simulink model "ADIA"  (R2018b)
settings: Solver=FixedStepDiscrete  StartTime=0.0  StopTime=10.0  FixedStep=0.02  RelTol=1e-3
undefined symbols (not defined in the file or in its folder): ACC_State_Active, ACC_State_BrakeOnly, ACC_State_Suspended, ACC_State_WaitingRise, ADAS_AEBBrakingProg, ADAS_DeclControlReq, ADAS_DriveOff, ADAS_ESCHoldReq_NotHold, ADASDecType_ACC, ADASDecType_AEB, ADIA_ACC_Acceleration_OOR_DecCount_C, ADIA_ACC_Acceleration_OOR_Duration_C, ADIA_ACC_Acceleration_OOR_IncCount_C, ADIA_ACC_Acceleration_OOR_LLim_C, ADIA_ACC_Acceleration_OOR_ULim_C, ADIA_ACC_AccelTrqReq_MixedDia_ULim_C, ADIA_ACC_AccelTrqReq_ULim_C, ADIA_ACC_Deceleration_Mixed_ULim_C, ADIA_ACC_Deceleration_OOR_DecCount_C, ADIA_ACC_Deceleration_OOR_Duration_C, ADIA_ACC_Deceleration_OOR_IncCount_C, ADIA_ACC_Deceleration_OOR_LLim_C, ADIA_ACC_Deceleration_OOR_ULim_C, ADIA_ACC_DriveOff_Distance_C, ADIA_ACC_DriveOff_TimeLim_C, ADIA_ACC_ReqMixed_DecCount_C, ADIA_ACC_ReqMixed_Duration_C, ADIA_ACC_ReqMixed_IncCount_C, ADIA_AccPedalRaw_MaxLim_C, ADIA_AccPedalRaw_MinLim_C, ADIA_ADAS_HoldDecReq_Set_C, ADIA_ADAS_HoldRConfirm_TimeLim_C, ADIA_ADAS_HoldVehSpd_Lim_C, ADIA_AEB_VehSpdDec_LLim_C, ADIA_AEB_VehSpdDec_ULim_C, ADIA_ASWFault_OvrdEn_C, ADIA_ASWFault_OvrdValue_C, ADIA_BatteryOutOfRange_DecCount_C, ADIA_BatteryOutOfRange_Duration_C, ADIA_BatteryOutOfRange_IncCount_C, ADIA_BattVolt_MaxLim_C, ADIA_BattVolt_MinLim_C, ADIA_BCM3_33C_InvBrkLight_DecCount_C, ADIA_BCM3_33C_InvBrkLight_Duration_C, ADIA_BCM3_33C_InvBrkLight_IncCount_C, ADIA_BCM_BattVolt_OvrdEn_C, ADIA_BCM_BattVolt_OvrdVal_C, ADIA_BCM_BrakeLampStaus_OvrdEn_C, ADIA_BCM_BrakeLampStaus_OvrdVal_C, ADIA_BCM_CHMSLStaus_OvrdEn_C, ADIA_BCM_CHMSLStaus_OvrdVal_C, ADIA_BCM_LeftTurnSwSt_OvrdEn_C, ADIA_BCM_LeftTurnSwSt_OvrdVal_C, ADIA_BCM_RightTurnSwSt_OvrdEn_C, ADIA_BCM_RightTurnSwSt_OvrdVal_C, ADIA_BCM_TurnSwFailure_DecCount_C, ADIA_BCM_TurnSwFailure_Duration_C, ADIA_BCM_TurnSwFailure_IncCount_C, ADIA_BSWFault_Ignore_C, ADIA_BSWFault_OvrdEn_C ... (+281)
libraries: simulink x208
(part 4 of 10)

== system ADIA/ADAS_Diagnostics/Diagnostics_Processing/DTC_ACC_Displacement_Safety_Violation ==
  note: may have some reset question
  ADIAve_y_ADAS_ESCDriveOff : Inport  OutDataTypeStr=UInt8  PortDimensions=1
  ADIAve_y_ADAS_ESCHoldReq : Inport  Port=2  OutDataTypeStr=UInt8  PortDimensions=1
  ADIAve_y_ADAS_ACCState : Inport  Port=3  OutDataTypeStr=UInt8  PortDimensions=1
  ADIAve_g_ESC_VehSpd : Inport  Port=4  OutDataTypeStr=single  PortDimensions=1
  Constant1 : Constant  Value=SYS_dT20ms
  Constant11 : Constant  Value=ADIA_ACC_DriveOff_TimeLim_C
  Constant12 : Constant  Value=ADIA_ACC_DriveOff_Distance_C
  Constant2 : Constant  Value=mps_to_kph  OutDataTypeStr=Inherit: Inherit via back propagation
  Constant3 : Constant  Value=ADAS_DriveOff
  Constant4 : Constant  Value=SYS_dT20ms
  Constant5 : Constant  Value=SYS_False
  Constant6 : Constant  Value=0
  Constant7 : Constant  Value=ADAS_ESCHoldReq_NotHold
  Constant9 : Constant  Value=ACC_State_Active  OutDataTypeStr=Inherit: Inherit via back propagation
  Counter : Subsystem
  Divide : Product  Inputs=*/
  Divide1 : Product  Inputs=**
  Latch 2 : Subsystem
  Logical Operator{1,3,7..8} (4 alike) : Logic  Operator=NOT  AllPortsSameDT=off  OutDataTypeStr=boolean
  Logical Operator{2,4..6} (4 alike) : Logic  AllPortsSameDT=off  OutDataTypeStr=boolean
  Relational Operator1 : RelationalOperator  Operator===  OutDataTypeStr=boolean  RndMeth=Simplest
  Relational Operator5 : RelationalOperator  Operator===  OutDataTypeStr=boolean  RndMeth=Simplest
  Relational Operator7 : RelationalOperator  Operator===  OutDataTypeStr=boolean  RndMeth=Simplest
  Terminator : Terminator
  Terminator1 : Terminator
  Timer1 : Subsystem
  ADIA_DTC_ACC_Displacement_Safety_Violation : Outport
  wires:
  ADIAve_y_ADAS_ESCHoldReq/1 -> Relational Operator5/1
  Constant7/1 -> Relational Operator5/2
  Relational Operator5/1 -> Logical Operator4/2
  Constant9/1 -> Relational Operator7/2
  ADIAve_y_ADAS_ACCState/1 -> Relational Operator7/1
  Relational Operator7/1 -> Logical Operator5/1
  Logical Operator5/1 -> Logical Operator3/1, Logical Operator2/2, Timer1/1(incrcondition)
  Constant12/1 -> Counter/2(maxlimit)
  Counter/2(counter_status) -> Logical Operator8/1, Latch 2/1(Input)
  Counter/1(counter out) -> Terminator/1
  Latch 2/1(Output) -> ADIA_DTC_ACC_Displacement_Safety_Violation/1
  ADIAve_g_ESC_VehSpd/1 -> Divide/1
  Constant2/1 -> Divide/2
  ADIAve_y_ADAS_ESCDriveOff/1 -> Relational Operator1/1
  Constant3/1 -> Relational Operator1/2
  Logical Operator4/1 -> Logical Operator5/2
  Relational Operator1/1 -> Logical Operator4/1
  Divide/1 -> Divide1/1
  Divide1/1 -> Counter/1(ADIAve_g_ESC_VeSpd)
  Constant4/1 -> Divide1/2
  Constant1/1 -> Timer1/2(incrvalue)
  Constant5/1 -> Timer1/3(decr condition)
  Constant6/1 -> Timer1/4(decvalue)
  Constant11/1 -> Timer1/5(maxlimit)
  Timer1/2(counter_status) -> Logical Operator1/1
  Logical Operator2/1 -> Logical Operator7/1, Counter/Enable
  Logical Operator1/1 -> Logical Operator2/1
  Timer1/1(counter out) -> Terminator1/1
  Logical Operator3/1 -> Timer1/6(reset)
  Logical Operator7/1 -> Logical Operator6/1
  Logical Operator6/1 -> Latch 2/2(Latch Reset)
  Logical Operator8/1 -> Logical Operator6/2

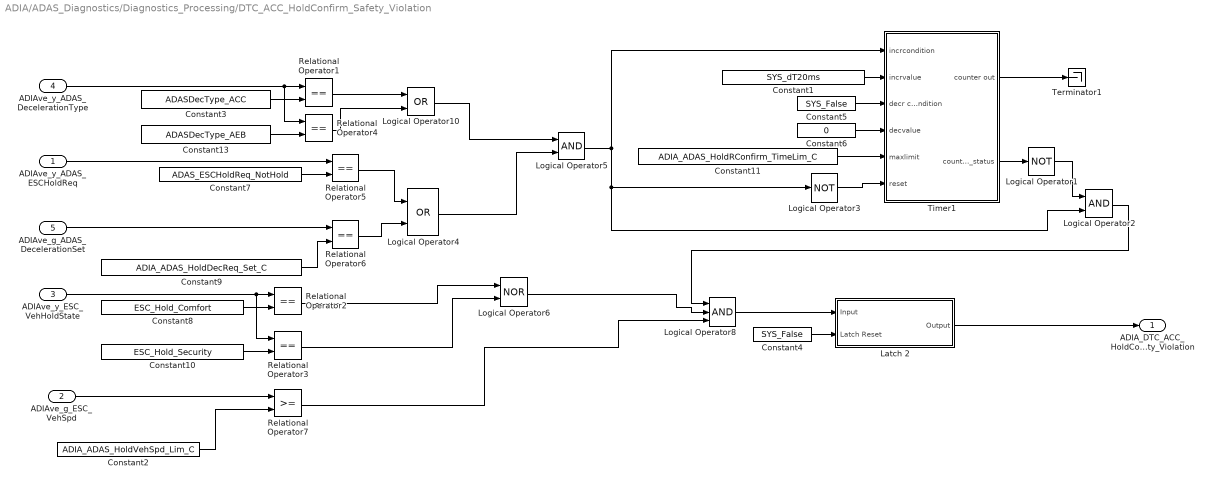
== system ADIA/ADAS_Diagnostics/Diagnostics_Processing/DTC_ACC_HoldConfirm_Safety_Violation ==
  ADIAve_y_ADAS_ESCHoldReq : Inport  OutDataTypeStr=UInt8  PortDimensions=1
  ADIAve_g_ESC_VehSpd : Inport  Port=2  OutDataTypeStr=single  PortDimensions=1
  ADIAve_y_ESC_VehHoldState : Inport  Port=3  OutDataTypeStr=uint8  PortDimensions=1
  ADIAve_y_ADAS_DecelerationType : Inport  Port=4  OutDataTypeStr=UInt8  PortDimensions=1
  ADIAve_g_ADAS_DecelerationSet : Inport  Port=5  OutDataTypeStr=T_M_Nm_Float32  PortDimensions=1
  Constant1 : Constant  Value=SYS_dT20ms
  Constant10 : Constant  Value=ESC_Hold_Security
  Constant11 : Constant  Value=ADIA_ADAS_HoldRConfirm_TimeLim_C
  Constant13 : Constant  Value=ADASDecType_AEB
  Constant2 : Constant  Value=ADIA_ADAS_HoldVehSpd_Lim_C
  Constant3 : Constant  Value=ADASDecType_ACC
  Constant4 : Constant  Value=SYS_False
  Constant5 : Constant  Value=SYS_False
  Constant6 : Constant  Value=0
  Constant7 : Constant  Value=ADAS_ESCHoldReq_NotHold
  Constant8 : Constant  Value=ESC_Hold_Comfort
  Constant9 : Constant  Value=ADIA_ADAS_HoldDecReq_Set_C
  Latch 2 : Subsystem
  Logical Operator1 : Logic  Operator=NOT  AllPortsSameDT=off  OutDataTypeStr=boolean
  Logical Operator10 : Logic  Operator=OR  AllPortsSameDT=off  OutDataTypeStr=boolean
  Logical Operator2 : Logic  AllPortsSameDT=off  OutDataTypeStr=boolean
  Logical Operator3 : Logic  Operator=NOT  AllPortsSameDT=off  OutDataTypeStr=boolean
  Logical Operator4 : Logic  Operator=OR  AllPortsSameDT=off  OutDataTypeStr=boolean
  Logical Operator5 : Logic  AllPortsSameDT=off  OutDataTypeStr=boolean
  Logical Operator6 : Logic  Operator=NOR  AllPortsSameDT=off  OutDataTypeStr=boolean
  Logical Operator8 : Logic  Inputs=3  AllPortsSameDT=off  OutDataTypeStr=boolean
  Relational Operator{1..6} (6 alike) : RelationalOperator  Operator===  OutDataTypeStr=boolean  RndMeth=Simplest
  Relational Operator7 : RelationalOperator  OutDataTypeStr=boolean  RndMeth=Simplest
  Terminator1 : Terminator
  Timer1 : Subsystem
  ADIA_DTC_ACC_HoldConfirm_Safety_Violation : Outport
  wires:
  Logical Operator3/1 -> Timer1/6(reset)
  Timer1/1(counter out) -> Terminator1/1
  Logical Operator1/1 -> Logical Operator2/1
  Logical Operator2/1 -> Logical Operator8/1
  Timer1/2(counter_status) -> Logical Operator1/1
  Constant11/1 -> Timer1/5(maxlimit)
  Constant6/1 -> Timer1/4(decvalue)
  Constant5/1 -> Timer1/3(decr condition)
  Constant1/1 -> Timer1/2(incrvalue)
  Logical Operator4/1 -> Logical Operator5/2
  Constant2/1 -> Relational Operator7/2
  ADIAve_g_ESC_VehSpd/1 -> Relational Operator7/1
  Latch 2/1(Output) -> ADIA_DTC_ACC_HoldConfirm_Safety_Violation/1
  Logical Operator5/1 -> Timer1/1(incrcondition), Logical Operator2/2, Logical Operator3/1
  Relational Operator5/1 -> Logical Operator4/1
  Constant7/1 -> Relational Operator5/2
  ADIAve_y_ADAS_ESCHoldReq/1 -> Relational Operator5/1
  ADIAve_y_ESC_VehHoldState/1 -> Relational Operator3/1, Relational Operator2/1
  Constant8/1 -> Relational Operator2/2
  Constant10/1 -> Relational Operator3/2
  Relational Operator3/1 -> Logical Operator6/2
  ADIAve_y_ADAS_DecelerationType/1 -> Relational Operator4/1, Relational Operator1/1
  Constant3/1 -> Relational Operator1/2
  Constant13/1 -> Relational Operator4/2
  Relational Operator1/1 -> Logical Operator10/1
  Relational Operator4/1 -> Logical Operator10/2
  ADIAve_g_ADAS_DecelerationSet/1 -> Relational Operator6/1
  Constant9/1 -> Relational Operator6/2
  Relational Operator6/1 -> Logical Operator4/2
  Logical Operator10/1 -> Logical Operator5/1
  Relational Operator2/1 -> Logical Operator6/1
  Relational Operator7/1 -> Logical Operator8/3
  Logical Operator6/1 -> Logical Operator8/2
  Logical Operator8/1 -> Latch 2/1(Input)
  Constant4/1 -> Latch 2/2(Latch Reset)

== system ADIA/ADAS_Diagnostics/Diagnostics_Processing/DTC_ACC_Mixed_Mode_Conflict ==
  ADIAve_y_ADAS_ACCState : Inport  OutDataTypeStr=UInt8  PortDimensions=1
  ADIAve_y_ADAS_DecelerationType : Inport  Port=2  OutDataTypeStr=UInt8  PortDimensions=1
  ADIAve_g_ADAS_ACCTorqueReq : Inport  Port=3  OutDataTypeStr=T_M_Nm_Float32  PortDimensions=1
  ADIAve_g_ADAS_DecelerationSet : Inport  Port=4  OutDataTypeStr=T_M_Nm_Float32  PortDimensions=1
  Constant : Constant  Value=ACC_State_Active
  Constant1 : Constant  Value=ACC_State_Suspended
  Constant2 : Constant  Value=ACC_State_WaitingRise
  Constant7 : Constant  Value=ACC_State_BrakeOnly
  Logical Operator4 : Logic  Operator=OR  Inputs=4  AllPortsSameDT=off  OutDataTypeStr=boolean
  Relational Operator{,1..2,5} (4 alike) : RelationalOperator  Operator===  OutDataTypeStr=boolean  RndMeth=Simplest
  Subsystem : Subsystem
  ADIA_DTC_ACC_Mixed_Mode_Conflict : Outport
  wires:
  Relational Operator5/1 -> Logical Operator4/2
  Constant7/1 -> Relational Operator5/2
  Relational Operator/1 -> Logical Operator4/1
  ADIAve_y_ADAS_ACCState/1 -> Relational Operator/1, Relational Operator2/1, Relational Operator1/1, Relational Operator5/1
  Constant/1 -> Relational Operator/2
  ADIAve_y_ADAS_DecelerationType/1 -> Subsystem/1(ADIAve_y_ADAS_DecelerationType)
  ADIAve_g_ADAS_ACCTorqueReq/1 -> Subsystem/2(ADIAve_g_ADAS_ACCTorqueReq)
  ADIAve_g_ADAS_DecelerationSet/1 -> Subsystem/3(ADIAve_g_ADAS_DecelerationSet)
  Subsystem/1(ADIA_DTC_ACC_Mixed_Mode_Conflic) -> ADIA_DTC_ACC_Mixed_Mode_Conflict/1
  Logical Operator4/1 -> Subsystem/Enable
  Constant1/1 -> Relational Operator1/2
  Relational Operator1/1 -> Logical Operator4/3
  Constant2/1 -> Relational Operator2/2
  Relational Operator2/1 -> Logical Operator4/4

== system ADIA/ADAS_Diagnostics/Diagnostics_Processing/DTC_AEB_Safety_Violation ==
  ADIAve_g_ESC_VehSpd : Inport  OutDataTypeStr=single  PortDimensions=1
  ADIAve_y_ADAS_DecelerationType : Inport  Port=2  OutDataTypeStr=UInt8  PortDimensions=1
  ADIAve_y_ADAS_DeclControlReq : Inport  Port=3  OutDataTypeStr=UInt8  PortDimensions=1
  ADIAve_y_ADAS_AEBBrakingProg : Inport  Port=4  OutDataTypeStr=UInt8  PortDimensions=1
  Add : Sum  Inputs=+-
  Constant1 : Constant  Value=ADIA_AEB_VehSpdDec_LLim_C
  Constant13 : Constant  Value=ADASDecType_AEB
  Constant2 : Constant  Value=ADIA_AEB_VehSpdDec_ULim_C
  Constant3 : Constant  Value=ADAS_AEBBrakingProg
  Constant7 : Constant  Value=ADAS_DeclControlReq
  Latch 1 : Subsystem
  Logical Operator1 : Logic  Operator=NOT  AllPortsSameDT=off  OutDataTypeStr=boolean
  Logical Operator2 : Logic  AllPortsSameDT=off  OutDataTypeStr=boolean
  Logical Operator3 : Logic  Operator=NOT  AllPortsSameDT=off  OutDataTypeStr=boolean
  Logical Operator4 : Logic  Inputs=3  AllPortsSameDT=off  OutDataTypeStr=boolean
  Logical Operator5 : Logic  AllPortsSameDT=off  OutDataTypeStr=boolean
  Relational Operator : RelationalOperator  Operator=>  OutDataTypeStr=boolean  RndMeth=Simplest
  Relational Operator1 : RelationalOperator  Operator===  OutDataTypeStr=boolean  RndMeth=Simplest
  Relational Operator2 : RelationalOperator  Operator=<=  OutDataTypeStr=boolean  RndMeth=Simplest
  Relational Operator4 : RelationalOperator  Operator===  OutDataTypeStr=boolean  RndMeth=Simplest
  Relational Operator5 : RelationalOperator  Operator===  OutDataTypeStr=boolean  RndMeth=Simplest
  Subsystem : Subsystem
  Subsystem1 : Subsystem
  Unit Delay : UnitDelay  SampleTime=-1
  Unit Delay1 : UnitDelay  SampleTime=-1
  DTC_AEB_Safety_Violation : Outport
  wires:
  Constant13/1 -> Relational Operator4/2
  ADIAve_y_ADAS_DecelerationType/1 -> Relational Operator4/1
  ADIAve_y_ADAS_DeclControlReq/1 -> Relational Operator5/1
  Constant7/1 -> Relational Operator5/2
  ADIAve_g_ESC_VehSpd/1 -> Subsystem1/1(ADIAve_g_ESC_VeSpd), Subsystem/1(ADIAve_g_ESC_VeSpd)
  Logical Operator4/1 -> Logical Operator3/1, Unit Delay1/1, Unit Delay/1, Logical Operator5/1
  Constant3/1 -> Relational Operator1/2
  ADIAve_y_ADAS_AEBBrakingProg/1 -> Relational Operator1/1
  Relational Operator1/1 -> Logical Operator4/3
  Relational Operator5/1 -> Logical Operator4/2
  Relational Operator4/1 -> Logical Operator4/1
  Logical Operator1/1 -> Logical Operator5/2
  Unit Delay/1 -> Logical Operator1/1
  Logical Operator5/1 -> Subsystem/Enable
  Unit Delay1/1 -> Logical Operator2/1
  Logical Operator3/1 -> Logical Operator2/2
  Logical Operator2/1 -> Subsystem1/Enable
  Subsystem/1(ADIA_AEB_Begin_VehSpd) -> Add/1
  Subsystem1/1(ADIA_AEB_End_VehSpd) -> Add/2
  Add/1 -> Relational Operator2/1, Relational Operator/1
  Constant2/1 -> Relational Operator/2
  Relational Operator/1 -> Latch 1/1(Input)
  Relational Operator2/1 -> Latch 1/2(Latch Reset)
  Latch 1/1(Output) -> DTC_AEB_Safety_Violation/1
  Constant1/1 -> Relational Operator2/2

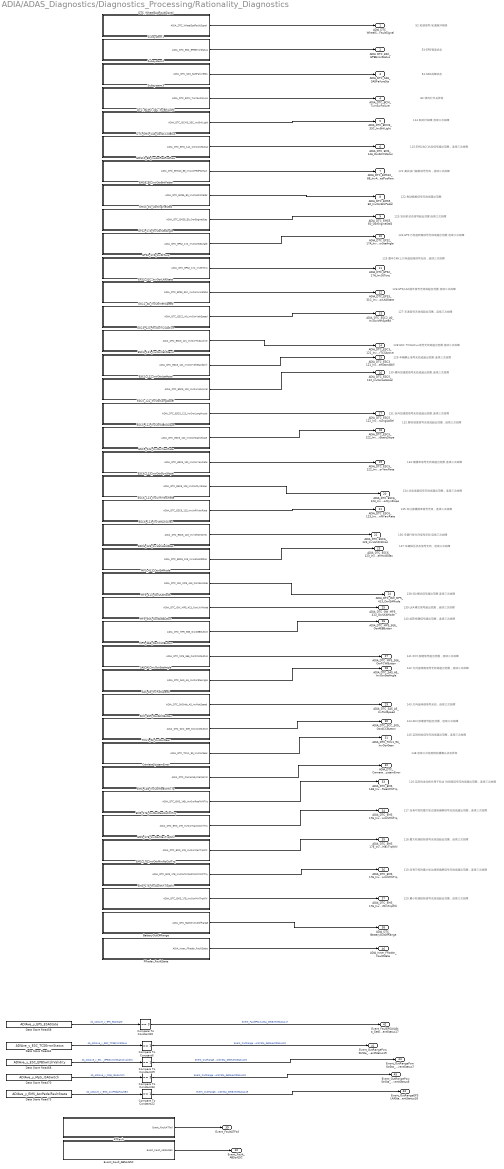
== system ADIA/ADAS_Diagnostics/Diagnostics_Processing/Rationality_Diagnostics ==
  note: 52:轮速信号/轮速脉冲错误
  note: 53:EPB错误状态
  note: 54:SAS故障状态
  note: 82:转向灯开关异常
  note: 114:制动灯故障,连续三次故障
  note: 115:EMS/ACC状态信号超出范围，连续三次故障
  note: 116:实际的发动机作用于轮边 的扭矩信号无效或超出范围，连续三次故障
  note: 117:没有可控的最大轮边扭矩偏移信号无效或超出范围，连续三次故障
  note: 118:最大轮端扭矩信号无效或超出范围，连续三次故障
  note: 119:没有可控的最小轮边扭矩偏移信号无效或超出范围，连续三次故障
  note: 120:最小轮端扭矩信号无效或超出范围，连续三次故障
  note: 121:真实油门踏板信号无效，连续三次故障
  note: 122:制动踏板信号无效或超出范围
  note: 123:发动机状态信号超出范围,连续三次故障
  note: 124:EPS 方向盘转角信号无效或超出范围,连续三次故障
  note: 125:整车CAN上方向盘扭矩信号无效，连续三次故障
  note: 126:EPS/LKA握手信号无效或超出范围,连续三次故障
  note: 127:车速信号无效或超出范围，连续三次故障
  note: 128:ESC TCSActive信号无效或超出范围,连续三次故障
  note: 129:车辆静止信号无效或超出范围,连续三次故障
  note: 130:横向加速度信号无效或超出范围,连续三次故障
  note: 131:纵向加速度信号无效或超出范围,连续三次故障
  note: 132:静态坡度信号无效或超出范围，连续三次故障
  note: 133:横摆率信号无效或超出范围,连续三次故障
  note: 134:动态坡度信号无效或超出范围，连续三次故障
  note: 135:未过滤横摆率信号无效，连续三次故障
  note: 136:车辆行驶方向信号无效,连续三次故障
  note: 137:车辆保压状态信号无效，连续三次故障
  note: 138:ISA模式信号超出范围,连续三次故障
  note: 139:LKA模式信号超出范围，连续三次故障
  note: 140:AEB按键信号超出范围，连续三次故障
  note: 141:FCW按键信号超出范围，连续三次故障
  note: 142:方向盘转角信号无效或超出范围，连续三次故障
  note: 143:方向盘转速信号无效，连续三次故障
  note: 144:ACC按键信号超出范围，连续三次故障
  note: 145:实际档位信号无效或超出范围，连续三次故障
  note: 148:连续三次检测到前摄像头状态异常
  ATFault : Subsystem
  BatteryOutOfRange : Subsystem
  CameraSystemError : Subsystem
  Compare To Constant20 : simulink/Logic and Bit Operations/Compare To Constant  relop===  const=3  OutDataTypeStr=boolean
  Compare To Constant22 : simulink/Logic and Bit Operations/Compare To Constant  relop===  const=1  OutDataTypeStr=boolean
  Compare To Constant29 : simulink/Logic and Bit Operations/Compare To Constant  relop===  const=1  OutDataTypeStr=boolean
  Compare To Constant33 : simulink/Logic and Bit Operations/Compare To Constant  relop===  const=3  OutDataTypeStr=boolean
  Compare To Constant6 : simulink/Logic and Bit Operations/Compare To Constant  relop===  const=1  OutDataTypeStr=boolean
  DTC_BCM3_33C_InvBrkLight : Subsystem
  DTC_EMS_14A_OorACCStatus : Subsystem
  DTC_WheelSpdFaultSignal : Subsystem
  Data Store Read58 : DataStoreRead  DataStoreName=ADIAve_y_EPS_ESAState
  Data Store Read62 : DataStoreRead  DataStoreName=ADIAve_y_ESC_TCSErrorStatus
  Data Store Read68 : DataStoreRead  DataStoreName=ADIAve_y_ESC_EPBSwitchValidity
  Data Store Read70 : DataStoreRead  DataStoreName=ADIAve_y_Mp5_ISASwitch
  Data Store Read73 : DataStoreRead  DataStoreName=ADIAve_y_EMS_AccPedalFaultState
  EMS10_88_InvAccPedPosRaw : Subsystem
  EMS5_E0_InvOorBrkPedal : Subsystem
  EMS5_E0_OorEngineStas : Subsystem
  EMS_14B_InvOorRealWhlTrq : Subsystem
  EMS_17E_InvOorMaxNoCtrlTrq : Subsystem
  EMS_17E_InvOorMaxTrqWhl : Subsystem
  EMS_17E_InvOorMinNoCtrlTrq : Subsystem
  EMS_17E_InvOorMinTrqWhl : Subsystem
  EPS2_17A_InvOorSteAngle : Subsystem
  EPS2_17A_InvStTorq : Subsystem
  EPS3_31C_InvOorLKAState : Subsystem
  ESC2_A0_InvOorVehSpeed : Subsystem
  ESC3_121_InvOorTCSActive : Subsystem
  ESC3_121_InvOorVehStand : Subsystem
  ESC5_122_InvOorLatAccel : Subsystem
  ESC5_122_InvOorLongiAccel : Subsystem
  ESC5_122_InvOorStaticSlope : Subsystem
  ESC5_122_InvOorYawRate : Subsystem
  ESC6_123_InvOorDynSlope : Subsystem
  ESC6_123_InvUnfilYawRate : Subsystem
  ESC6_123_InvVehDriDirec : Subsystem
  ESC6_123_InvVehHoldStas : Subsystem
  Event_Fault_ABSorESC : Subsystem
  FRadar_FaultState : Subsystem
  MP5_366_OorAEBButton : Subsystem
  MP5_366_OorFCWButton : Subsystem
  MP5_413_OorISAMode : Subsystem
  MP5_413_OorLKAMode : Subsystem
  SAS_A5_InvOorSteAngle : Subsystem
  SAS_A5_InvRotSpeed : Subsystem
  SCC_309_OorACCButton : Subsystem
  Subsystem1 : Subsystem
  Subsystem2 : Subsystem
  Subsystem3 : Subsystem
  TCU1_93_InvOorGear : Subsystem
  ADIA_DTC_WheelSpdFaultSignal : Outport
  ADIA_DTC_ESC_EPBErrorStatus : Outport  Port=2
  ADIA_DTC_SAS_SASFailureSts : Outport  Port=3
  ADIA_DTC_BCM_TurnSwFailure : Outport  Port=4
  ADIA_DTC_BCM3_33C_InvBrkLight : Outport  Port=5
  ADIA_DTC_EMS_14A_OorACCStatus : Outport  Port=6
  ADIA_DTC_EMS10_88_InvAccPedPosRaw : Outport  Port=7
  ADIA_DTC_EMS5_E0_InvOorBrkPedal : Outport  Port=8
  ADIA_DTC_EMS5_E0_OorEngineStas : Outport  Port=9
  ADIA_DTC_EPS2_17A_InvOorSteAngle : Outport  Port=10
  ADIA_DTC_EPS2_17A_InvStTorq : Outport  Port=11
  ADIA_DTC_EPS3_31C_InvOorLKAState : Outport  Port=12
  ADIA_DTC_ESC2_A0_InvOorVehSpeed : Outport  Port=13
  ADIA_DTC_ESC3_121_InvOorTCSActive : Outport  Port=14
  ADIA_DTC_ESC3_121_InvOorVehStandstill : Outport  Port=15
  ADIA_DTC_ESC5_122_InvOorLatAccel : Outport  Port=16
  ADIA_DTC_ESC5_122_InvOorLongiAccel : Outport  Port=17
  ADIA_DTC_ESC5_122_InvOorStaticSlope : Outport  Port=18
  ADIA_DTC_ESC5_122_InvOorYawRate : Outport  Port=19
  ADIA_DTC_ESC6_123_InvOorDynSlope : Outport  Port=20
  ADIA_DTC_ESC6_123_InvUnfilYawRate : Outport  Port=21
  ADIA_DTC_ESC6_123_InvVehDriDirec : Outport  Port=22
  ADIA_DTC_ESC6_123_InvVehHoldStas : Outport  Port=23
  ADIA_DTC_GW_MP5_413_OorISAMode : Outport  Port=24
  ADIA_DTC_GW_MP5_413_OorLKAMode : Outport  Port=25
  ADIA_DTC_MP5_366_OorAEBButton : Outport  Port=26
  ADIA_DTC_MP5_366_OorFCWButton : Outport  Port=27
  ADIA_DTC_SAS_A5_InvOorSteAngle : Outport  Port=28
  ADIA_DTC_SAS_A5_InvRotSpeed : Outport  Port=29
  ADIA_DTC_SCC_309_OorACCButton : Outport  Port=30
  ADIA_DTC_TCU1_93_InvOorGear : Outport  Port=31
  ADIA_DTC_CameraSystemError : Outport  Port=32
  ADIA_DTC_EMS_14B_InvOorRealWhlTrq : Outport  Port=33
  ADIA_DTC_EMS_17E_InvOorMaxNotContrlWhlTrq : Outport  Port=34
  ADIA_DTC_EMS_17E_InvOorMaxTrqWhl : Outport  Port=35
  ADIA_DTC_EMS_17E_InvOorMinNotContrlWhlTrq : Outport  Port=36
  ADIA_DTC_EMS_17E_InvOorMinTrqWhl : Outport  Port=37
  ADIA_DTC_BatteryOutOfRange : Outport  Port=38
  Event_FaultATFail : Outport  Port=39
  "Event_Fault_ABSorESC " : Outport  Port=40
  Event_OutRangePowStrSta_SetEventStatus19 : Outport  Port=41
  Event_FaulEPSLKASta_SetEventStatus17 : Outport  Port=42
  Event_OutRangeEPSLKASta_SetEventStatus18 : Outport  Port=43
  Event_OutRangePowStrSta_SetEventStatus7 : Outport  Port=44
  Event_OutRangePowStrSta_SetEventStatus9 : Outport  Port=45
  ADIA_Inner_FRadar_FaultState : Outport  Port=46
  wires:
  Data Store Read58/1 -> Compare To Constant20/1  "ob_ADIAve_y_EPS_ESAState"
  Data Store Read62/1 -> Compare To Constant6/1  "ob_ADIAve_y_ESC_TCSErrorStatus"
  Data Store Read70/1 -> Compare To Constant33/1  "ob_ADIAve_y_Mp5_ISASwitch"
  Data Store Read68/1 -> Compare To Constant29/1  "ob_ADIAve_y_ESC_EPBSwitchStaticsValidity"
  Compare To Constant6/1 -> Event_OutRangePowStrSta_SetEventStatus19/1  "Event_OutRangePowStrSta_SetEventStatus19"
  Compare To Constant29/1 -> Event_OutRangePowStrSta_SetEventStatus7/1  "Event_OutRangePowStrSta_SetEventStatus19"
  Compare To Constant20/1 -> Event_FaulEPSLKASta_SetEventStatus17/1  "Event_FaulEPSLKASta_SetEventStatus17"
  Compare To Constant33/1 -> Event_OutRangePowStrSta_SetEventStatus9/1  "Event_OutRangePowStrSta_SetEventStatus19"
  Data Store Read73/1 -> Compare To Constant22/1  "ob_ADIAve_y_EMS_AccPedalFaultBit"
  Compare To Constant22/1 -> Event_OutRangeEPSLKASta_SetEventStatus18/1  "Event_OutRangePowStrSta_SetEventStatus19"
  DTC_WheelSpdFaultSignal/1(ADIA_DTC_WheelSpdFaultSignal) -> ADIA_DTC_WheelSpdFaultSignal/1
  Event_Fault_ABSorESC/1("Event_Fault_ABSorESC ") -> "Event_Fault_ABSorESC "/1
  ATFault/1(Event_FaultATFail) -> Event_FaultATFail/1
  DTC_BCM3_33C_InvBrkLight/1(ADIA_DTC_BCM3_33C_InvBrkLight) -> ADIA_DTC_BCM3_33C_InvBrkLight/1
  DTC_EMS_14A_OorACCStatus/1(ADIA_DTC_EMS_14A_OorACCStatus) -> ADIA_DTC_EMS_14A_OorACCStatus/1
  EMS5_E0_OorEngineStas/1(ADIA_DTC_EMS5_E0_OorEngineStas) -> ADIA_DTC_EMS5_E0_OorEngineStas/1
  Subsystem1/1(ADIA_DTC_ESC_EPBErrorStatus) -> ADIA_DTC_ESC_EPBErrorStatus/1
  Subsystem2/1(ADIA_DTC_SAS_SASFailureSts) -> ADIA_DTC_SAS_SASFailureSts/1
  Subsystem3/1(ADIA_DTC_BCM_TurnSwFailure) -> ADIA_DTC_BCM_TurnSwFailure/1
  EMS10_88_InvAccPedPosRaw/1(ADIA_DTC_EMS10_88_InvAccPedPosRaw) -> ADIA_DTC_EMS10_88_InvAccPedPosRaw/1
  EMS5_E0_InvOorBrkPedal/1(ADIA_DTC_EMS5_E0_InvOorBrkPedal) -> ADIA_DTC_EMS5_E0_InvOorBrkPedal/1
  EPS2_17A_InvOorSteAngle/1(ADIA_DTC_EPS2_17A_InvOorSteAngle) -> ADIA_DTC_EPS2_17A_InvOorSteAngle/1
  EPS2_17A_InvStTorq/1(ADIA_DTC_EPS2_17A_InvStTorq) -> ADIA_DTC_EPS2_17A_InvStTorq/1
  EPS3_31C_InvOorLKAState/1(ADIA_DTC_EPS3_31C_InvOorLKAState) -> ADIA_DTC_EPS3_31C_InvOorLKAState/1
  ESC2_A0_InvOorVehSpeed/1(ADIA_DTC_ESC2_A0_InvOorVehSpeed) -> ADIA_DTC_ESC2_A0_InvOorVehSpeed/1
  ESC3_121_InvOorTCSActive/1(ADIA_DTC_ESC3_121_InvOorTCSActive) -> ADIA_DTC_ESC3_121_InvOorTCSActive/1
  ESC3_121_InvOorVehStand/1(ADIA_DTC_ESC3_121_InvOorVehStandstill) -> ADIA_DTC_ESC3_121_InvOorVehStandstill/1
  ESC5_122_InvOorLatAccel/1(ADIA_DTC_ESC5_122_InvOorLatAccel) -> ADIA_DTC_ESC5_122_InvOorLatAccel/1
  ESC5_122_InvOorLongiAccel/1(ADIA_DTC_ESC5_122_InvOorLongiAccel) -> ADIA_DTC_ESC5_122_InvOorLongiAccel/1
  ESC5_122_InvOorStaticSlope/1(ADIA_DTC_ESC5_122_InvOorStaticSlope) -> ADIA_DTC_ESC5_122_InvOorStaticSlope/1
  ESC5_122_InvOorYawRate/1(ADIA_DTC_ESC5_122_InvOorYawRate) -> ADIA_DTC_ESC5_122_InvOorYawRate/1
  ESC6_123_InvOorDynSlope/1(ADIA_DTC_ESC6_123_InvOorDynSlope) -> ADIA_DTC_ESC6_123_InvOorDynSlope/1
  ESC6_123_InvUnfilYawRate/1(ADIA_DTC_ESC6_123_InvUnfilYawRate) -> ADIA_DTC_ESC6_123_InvUnfilYawRate/1
  ESC6_123_InvVehDriDirec/1(ADIA_DTC_ESC6_123_InvVehDriDirec) -> ADIA_DTC_ESC6_123_InvVehDriDirec/1
  ESC6_123_InvVehHoldStas/1(ADIA_DTC_ESC6_123_InvVehHoldStas) -> ADIA_DTC_ESC6_123_InvVehHoldStas/1
  MP5_413_OorISAMode/1(ADIA_DTC_GW_MP5_413_OorISAMode) -> ADIA_DTC_GW_MP5_413_OorISAMode/1
  MP5_413_OorLKAMode/1(ADIA_DTC_GW_MP5_413_OorLKAMode) -> ADIA_DTC_GW_MP5_413_OorLKAMode/1
  MP5_366_OorAEBButton/1(ADIA_DTC_MP5_366_OorAEBButton) -> ADIA_DTC_MP5_366_OorAEBButton/1
  MP5_366_OorFCWButton/1(ADIA_DTC_MP5_366_OorFCWButton) -> ADIA_DTC_MP5_366_OorFCWButton/1
  SAS_A5_InvOorSteAngle/1(ADIA_DTC_SAS_A5_InvOorSteAngle) -> ADIA_DTC_SAS_A5_InvOorSteAngle/1
  SAS_A5_InvRotSpeed/1(ADIA_DTC_SASInfo_A5_InvRotSpeed) -> ADIA_DTC_SAS_A5_InvRotSpeed/1
  SCC_309_OorACCButton/1(ADIA_DTC_SCC_309_OorACCButton) -> ADIA_DTC_SCC_309_OorACCButton/1
  TCU1_93_InvOorGear/1(ADIA_DTC_TCU1_93_InvOorGear) -> ADIA_DTC_TCU1_93_InvOorGear/1
  CameraSystemError/1(ADIA_DTC_CameraSystemError) -> ADIA_DTC_CameraSystemError/1
  EMS_14B_InvOorRealWhlTrq/1(ADIA_DTC_EMS_14B_InvOorRealWhlTrq) -> ADIA_DTC_EMS_14B_InvOorRealWhlTrq/1
  EMS_17E_InvOorMaxNoCtrlTrq/1(ADIA_DTC_EMS_17E_InvOorMaxNoCtrlTrq) -> ADIA_DTC_EMS_17E_InvOorMaxNotContrlWhlTrq/1
  EMS_17E_InvOorMinNoCtrlTrq/1(ADIA_DTC_EMS_17E_InvOorMinNotContrlWhlTrq) -> ADIA_DTC_EMS_17E_InvOorMinNotContrlWhlTrq/1
  EMS_17E_InvOorMaxTrqWhl/1(ADIA_DTC_EMS_17E_InvOorMaxTrqWhl) -> ADIA_DTC_EMS_17E_InvOorMaxTrqWhl/1
  EMS_17E_InvOorMinTrqWhl/1(ADIA_DTC_EMS_17E_InvOorMinTrqWhl) -> ADIA_DTC_EMS_17E_InvOorMinTrqWhl/1
  BatteryOutOfRange/1("ADIA_DTC_BatteryOutOfRange ") -> ADIA_DTC_BatteryOutOfRange/1
  FRadar_FaultState/1(ADIA_Inner_FRadar_FaultState) -> ADIA_Inner_FRadar_FaultState/1

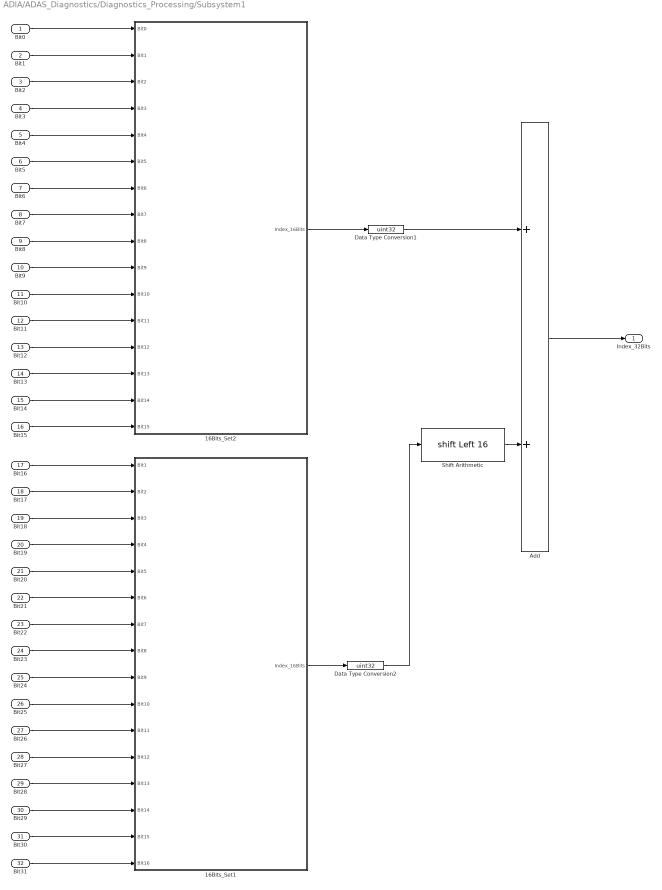
== system ADIA/ADAS_Diagnostics/Diagnostics_Processing/Subsystem1 ==
  Bit0 : Inport  OutDataTypeStr=boolean
  Bit1 : Inport  Port=2  OutDataTypeStr=boolean
  Bit2 : Inport  Port=3  OutDataTypeStr=boolean
  Bit3 : Inport  Port=4  OutDataTypeStr=boolean
  Bit4 : Inport  Port=5  OutDataTypeStr=boolean
  Bit5 : Inport  Port=6  OutDataTypeStr=boolean
  Bit6 : Inport  Port=7  OutDataTypeStr=boolean
  Bit7 : Inport  Port=8  OutDataTypeStr=boolean
  Bit8 : Inport  Port=9  OutDataTypeStr=boolean
  Bit9 : Inport  Port=10  OutDataTypeStr=boolean
  Bit10 : Inport  Port=11  OutDataTypeStr=boolean
  Bit11 : Inport  Port=12  OutDataTypeStr=boolean
  Bit12 : Inport  Port=13  OutDataTypeStr=boolean
  Bit13 : Inport  Port=14  OutDataTypeStr=boolean
  Bit14 : Inport  Port=15  OutDataTypeStr=boolean
  Bit15 : Inport  Port=16  OutDataTypeStr=boolean
  Bit16 : Inport  Port=17  OutDataTypeStr=boolean
  Bit17 : Inport  Port=18  OutDataTypeStr=boolean
  Bit18 : Inport  Port=19  OutDataTypeStr=boolean
  Bit19 : Inport  Port=20  OutDataTypeStr=boolean
  Bit20 : Inport  Port=21  OutDataTypeStr=boolean
  Bit21 : Inport  Port=22  OutDataTypeStr=boolean
  Bit22 : Inport  Port=23  OutDataTypeStr=boolean
  Bit23 : Inport  Port=24  OutDataTypeStr=boolean
  Bit24 : Inport  Port=25  OutDataTypeStr=boolean
  Bit25 : Inport  Port=26  OutDataTypeStr=boolean
  Bit26 : Inport  Port=27  OutDataTypeStr=boolean
  Bit27 : Inport  Port=28  OutDataTypeStr=boolean
  Bit28 : Inport  Port=29  OutDataTypeStr=boolean
  Bit29 : Inport  Port=30  OutDataTypeStr=boolean
  Bit30 : Inport  Port=31  OutDataTypeStr=boolean
  Bit31 : Inport  Port=32  OutDataTypeStr=boolean
  16Bits_Set1 : Subsystem
  16Bits_Set2 : Subsystem
  Add : Sum
  Data Type Conversion1 : DataTypeConversion  OutDataTypeStr=uint32
  Data Type Conversion2 : DataTypeConversion  OutDataTypeStr=uint32
  Shift Arithmetic : ArithShift  BitShiftNumber=16  BitShiftDirection=Left
  Index_32Bits : Outport
  wires:
  16Bits_Set2/1(Index_16Bits) -> Data Type Conversion1/1
  16Bits_Set1/1(Index_16Bits) -> Data Type Conversion2/1
  Data Type Conversion2/1 -> Shift Arithmetic/1
  Data Type Conversion1/1 -> Add/1
  Add/1 -> Index_32Bits/1
  Shift Arithmetic/1 -> Add/2
  Bit0/1 -> 16Bits_Set2/1(Bit0)
  Bit1/1 -> 16Bits_Set2/2(Bit1)
  Bit2/1 -> 16Bits_Set2/3(Bit2)
  Bit3/1 -> 16Bits_Set2/4(Bit3)
  Bit4/1 -> 16Bits_Set2/5(Bit4)
  Bit5/1 -> 16Bits_Set2/6(Bit5)
  Bit6/1 -> 16Bits_Set2/7(Bit6)
  Bit7/1 -> 16Bits_Set2/8(Bit7)
  Bit8/1 -> 16Bits_Set2/9(Bit8)
  Bit9/1 -> 16Bits_Set2/10(Bit9)
  Bit10/1 -> 16Bits_Set2/11(Bit10)
  Bit11/1 -> 16Bits_Set2/12(Bit11)
  Bit12/1 -> 16Bits_Set2/13(Bit12)
  Bit13/1 -> 16Bits_Set2/14(Bit13)
  Bit14/1 -> 16Bits_Set2/15(Bit14)
  Bit15/1 -> 16Bits_Set2/16(Bit15)
  Bit16/1 -> 16Bits_Set1/1(Bit1)
  Bit17/1 -> 16Bits_Set1/2(Bit2)
  Bit18/1 -> 16Bits_Set1/3(Bit3)
  Bit19/1 -> 16Bits_Set1/4(Bit4)
  Bit20/1 -> 16Bits_Set1/5(Bit5)
  Bit21/1 -> 16Bits_Set1/6(Bit6)
  Bit22/1 -> 16Bits_Set1/7(Bit7)
  Bit23/1 -> 16Bits_Set1/8(Bit8)
  Bit24/1 -> 16Bits_Set1/9(Bit9)
  Bit25/1 -> 16Bits_Set1/10(Bit10)
  Bit26/1 -> 16Bits_Set1/11(Bit11)
  Bit27/1 -> 16Bits_Set1/12(Bit12)
  Bit28/1 -> 16Bits_Set1/13(Bit13)
  Bit29/1 -> 16Bits_Set1/14(Bit14)
  Bit30/1 -> 16Bits_Set1/15(Bit15)
  Bit31/1 -> 16Bits_Set1/16(Bit16)

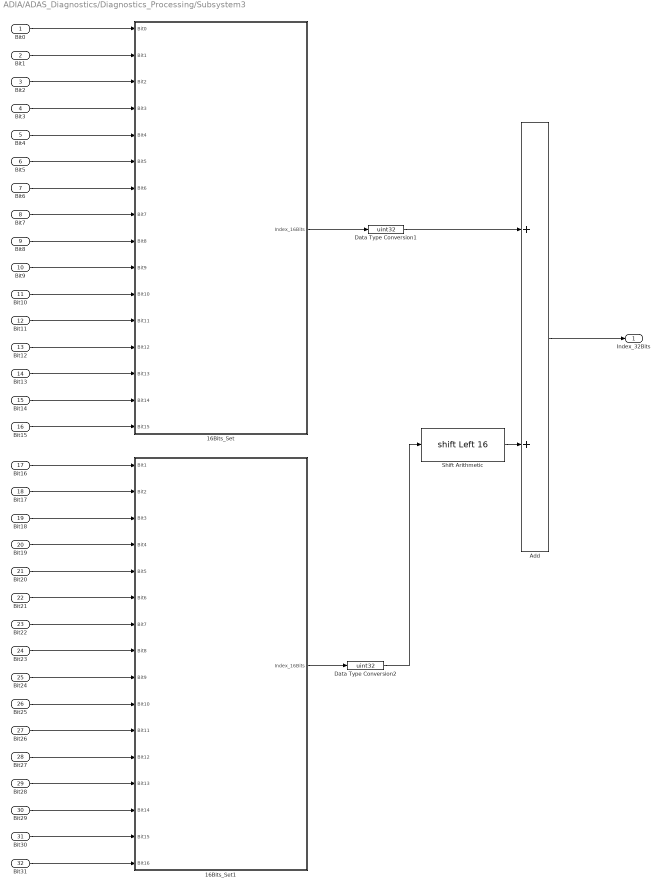
== system ADIA/ADAS_Diagnostics/Diagnostics_Processing/Subsystem3 ==
  Bit0 : Inport  OutDataTypeStr=boolean
  Bit1 : Inport  Port=2  OutDataTypeStr=boolean
  Bit2 : Inport  Port=3  OutDataTypeStr=boolean
  Bit3 : Inport  Port=4  OutDataTypeStr=boolean
  Bit4 : Inport  Port=5  OutDataTypeStr=boolean
  Bit5 : Inport  Port=6  OutDataTypeStr=boolean
  Bit6 : Inport  Port=7  OutDataTypeStr=boolean
  Bit7 : Inport  Port=8  OutDataTypeStr=boolean
  Bit8 : Inport  Port=9  OutDataTypeStr=boolean
  Bit9 : Inport  Port=10  OutDataTypeStr=boolean
  Bit10 : Inport  Port=11  OutDataTypeStr=boolean
  Bit11 : Inport  Port=12  OutDataTypeStr=boolean
  Bit12 : Inport  Port=13  OutDataTypeStr=boolean
  Bit13 : Inport  Port=14  OutDataTypeStr=boolean
  Bit14 : Inport  Port=15  OutDataTypeStr=boolean
  Bit15 : Inport  Port=16  OutDataTypeStr=boolean
  Bit16 : Inport  Port=17  OutDataTypeStr=boolean
  Bit17 : Inport  Port=18  OutDataTypeStr=boolean
  Bit18 : Inport  Port=19  OutDataTypeStr=boolean
  Bit19 : Inport  Port=20  OutDataTypeStr=boolean
  Bit20 : Inport  Port=21  OutDataTypeStr=boolean
  Bit21 : Inport  Port=22  OutDataTypeStr=boolean
  Bit22 : Inport  Port=23  OutDataTypeStr=boolean
  Bit23 : Inport  Port=24  OutDataTypeStr=boolean
  Bit24 : Inport  Port=25  OutDataTypeStr=boolean
  Bit25 : Inport  Port=26  OutDataTypeStr=boolean
  Bit26 : Inport  Port=27  OutDataTypeStr=boolean
  Bit27 : Inport  Port=28  OutDataTypeStr=boolean
  Bit28 : Inport  Port=29  OutDataTypeStr=boolean
  Bit29 : Inport  Port=30  OutDataTypeStr=boolean
  Bit30 : Inport  Port=31  OutDataTypeStr=boolean
  Bit31 : Inport  Port=32  OutDataTypeStr=boolean
  16Bits_Set : Subsystem
  16Bits_Set1 : Subsystem
  Add : Sum
  Data Type Conversion1 : DataTypeConversion  OutDataTypeStr=uint32
  Data Type Conversion2 : DataTypeConversion  OutDataTypeStr=uint32
  Shift Arithmetic : ArithShift  BitShiftNumber=16  BitShiftDirection=Left
  Index_32Bits : Outport
  wires:
  Bit31/1 -> 16Bits_Set1/16(Bit16)
  Bit30/1 -> 16Bits_Set1/15(Bit15)
  Bit29/1 -> 16Bits_Set1/14(Bit14)
  Bit28/1 -> 16Bits_Set1/13(Bit13)
  Bit27/1 -> 16Bits_Set1/12(Bit12)
  Bit26/1 -> 16Bits_Set1/11(Bit11)
  Bit25/1 -> 16Bits_Set1/10(Bit10)
  Bit24/1 -> 16Bits_Set1/9(Bit9)
  Bit23/1 -> 16Bits_Set1/8(Bit8)
  Bit22/1 -> 16Bits_Set1/7(Bit7)
  Bit21/1 -> 16Bits_Set1/6(Bit6)
  Bit20/1 -> 16Bits_Set1/5(Bit5)
  Bit19/1 -> 16Bits_Set1/4(Bit4)
  Bit18/1 -> 16Bits_Set1/3(Bit3)
  Bit17/1 -> 16Bits_Set1/2(Bit2)
  Bit16/1 -> 16Bits_Set1/1(Bit1)
  Bit15/1 -> 16Bits_Set/16(Bit15)
  Bit14/1 -> 16Bits_Set/15(Bit14)
  Bit13/1 -> 16Bits_Set/14(Bit13)
  Bit12/1 -> 16Bits_Set/13(Bit12)
  Bit11/1 -> 16Bits_Set/12(Bit11)
  Bit10/1 -> 16Bits_Set/11(Bit10)
  Bit9/1 -> 16Bits_Set/10(Bit9)
  Bit8/1 -> 16Bits_Set/9(Bit8)
  Bit7/1 -> 16Bits_Set/8(Bit7)
  Bit6/1 -> 16Bits_Set/7(Bit6)
  Bit5/1 -> 16Bits_Set/6(Bit5)
  Bit4/1 -> 16Bits_Set/5(Bit4)
  Bit3/1 -> 16Bits_Set/4(Bit3)
  Bit2/1 -> 16Bits_Set/3(Bit2)
  Bit1/1 -> 16Bits_Set/2(Bit1)
  Bit0/1 -> 16Bits_Set/1(Bit0)
  Shift Arithmetic/1 -> Add/2
  Add/1 -> Index_32Bits/1
  Data Type Conversion1/1 -> Add/1
  Data Type Conversion2/1 -> Shift Arithmetic/1
  16Bits_Set1/1(Index_16Bits) -> Data Type Conversion2/1
  16Bits_Set/1(Index_16Bits) -> Data Type Conversion1/1

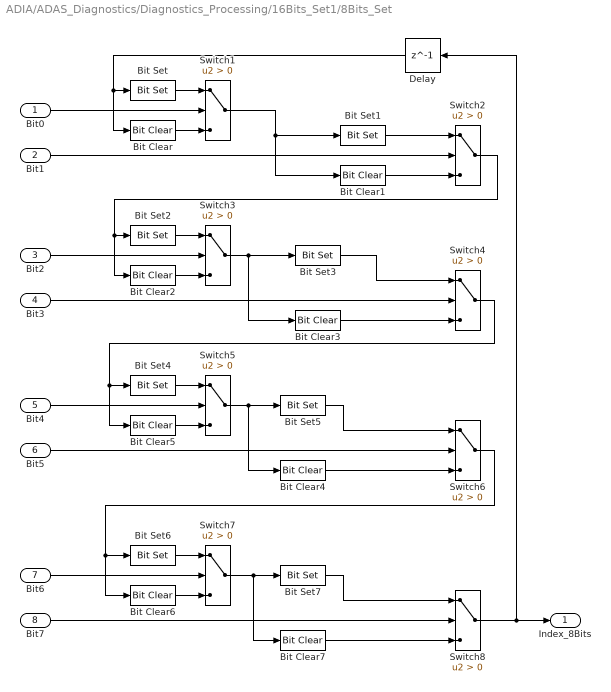
== system ADIA/ADAS_Diagnostics/Diagnostics_Processing/16Bits_Set1/8Bits_Set ==
  Bit0 : Inport  OutDataTypeStr=boolean
  Bit1 : Inport  Port=2  OutDataTypeStr=boolean
  Bit2 : Inport  Port=3  OutDataTypeStr=boolean
  Bit3 : Inport  Port=4  OutDataTypeStr=boolean
  Bit4 : Inport  Port=5  OutDataTypeStr=boolean
  Bit5 : Inport  Port=6  OutDataTypeStr=boolean
  Bit6 : Inport  Port=7  OutDataTypeStr=boolean
  Bit7 : Inport  Port=8  OutDataTypeStr=boolean
  Bit Clear : simulink/Logic and Bit Operations/Bit Clear  iBit=0
      settings: SourceProductName=Simulink  SourceProductBaseCode=SL
  Bit Clear1 : simulink/Logic and Bit Operations/Bit Clear  iBit=1
      settings: SourceProductName=Simulink  SourceProductBaseCode=SL
  Bit Clear2 : simulink/Logic and Bit Operations/Bit Clear  iBit=2
      settings: SourceProductName=Simulink  SourceProductBaseCode=SL
  Bit Clear3 : simulink/Logic and Bit Operations/Bit Clear  iBit=3
      settings: SourceProductName=Simulink  SourceProductBaseCode=SL
  Bit Clear4 : simulink/Logic and Bit Operations/Bit Clear  iBit=5
      settings: SourceProductName=Simulink  SourceProductBaseCode=SL
  Bit Clear5 : simulink/Logic and Bit Operations/Bit Clear  iBit=4
      settings: SourceProductName=Simulink  SourceProductBaseCode=SL
  Bit Clear6 : simulink/Logic and Bit Operations/Bit Clear  iBit=6
      settings: SourceProductName=Simulink  SourceProductBaseCode=SL
  Bit Clear7 : simulink/Logic and Bit Operations/Bit Clear  iBit=7
      settings: SourceProductName=Simulink  SourceProductBaseCode=SL
  Bit Set : simulink/Logic and Bit Operations/Bit Set  iBit=0
      settings: SourceProductName=Simulink  SourceProductBaseCode=SL
  Bit Set1 : simulink/Logic and Bit Operations/Bit Set  iBit=1
      settings: SourceProductName=Simulink  SourceProductBaseCode=SL
  Bit Set2 : simulink/Logic and Bit Operations/Bit Set  iBit=2
      settings: SourceProductName=Simulink  SourceProductBaseCode=SL
  Bit Set3 : simulink/Logic and Bit Operations/Bit Set  iBit=3
      settings: SourceProductName=Simulink  SourceProductBaseCode=SL
  Bit Set4 : simulink/Logic and Bit Operations/Bit Set  iBit=4
      settings: SourceProductName=Simulink  SourceProductBaseCode=SL
  Bit Set5 : simulink/Logic and Bit Operations/Bit Set  iBit=5
      settings: SourceProductName=Simulink  SourceProductBaseCode=SL
  Bit Set6 : simulink/Logic and Bit Operations/Bit Set  iBit=6
      settings: SourceProductName=Simulink  SourceProductBaseCode=SL
  Bit Set7 : simulink/Logic and Bit Operations/Bit Set  iBit=7
      settings: SourceProductName=Simulink  SourceProductBaseCode=SL
  Delay : Delay  DelayLength=1  InitialCondition=0
  Switch{1..8} (8 alike) : Switch  Criteria=u2 > Threshold
  Index_8Bits : Outport  OutDataTypeStr=uint8
  wires:
  Bit Set7/1 -> Switch8/1
  Bit0/1 -> Switch1/2
  Bit3/1 -> Switch4/2
  Switch8/1 -> Index_8Bits/1, Delay/1
  Switch1/1 -> Bit Clear1/1, Bit Set1/1
  Bit1/1 -> Switch2/2
  Switch5/1 -> Bit Clear4/1, Bit Set5/1
  Delay/1 -> Bit Clear/1, Bit Set/1
  Bit Set1/1 -> Switch2/1
  Bit2/1 -> Switch3/2
  Bit5/1 -> Switch6/2
  Bit4/1 -> Switch5/2
  Bit Set6/1 -> Switch7/1
  Bit7/1 -> Switch8/2
  Bit6/1 -> Switch7/2
  Switch3/1 -> Bit Clear3/1, Bit Set3/1
  Bit Set/1 -> Switch1/1
  Bit Set3/1 -> Switch4/1
  Switch2/1 -> Bit Clear2/1, Bit Set2/1
  Switch7/1 -> Bit Clear7/1, Bit Set7/1
  Bit Set5/1 -> Switch6/1
  Switch6/1 -> Bit Clear6/1, Bit Set6/1
  Switch4/1 -> Bit Clear5/1, Bit Set4/1
  Bit Set2/1 -> Switch3/1
  Bit Set4/1 -> Switch5/1
  Bit Clear/1 -> Switch1/3
  Bit Clear1/1 -> Switch2/3
  Bit Clear2/1 -> Switch3/3
  Bit Clear3/1 -> Switch4/3
  Bit Clear4/1 -> Switch6/3
  Bit Clear5/1 -> Switch5/3
  Bit Clear6/1 -> Switch7/3
  Bit Clear7/1 -> Switch8/3

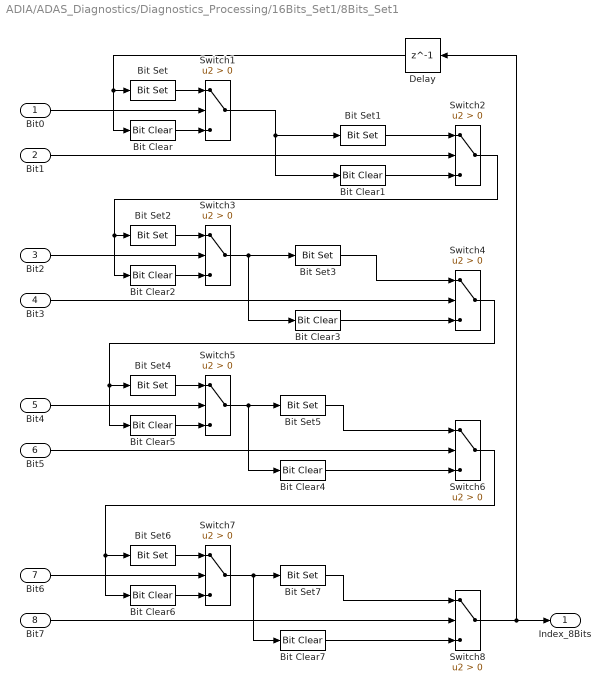
== system ADIA/ADAS_Diagnostics/Diagnostics_Processing/16Bits_Set1/8Bits_Set1 ==
  Bit0 : Inport  OutDataTypeStr=boolean
  Bit1 : Inport  Port=2  OutDataTypeStr=boolean
  Bit2 : Inport  Port=3  OutDataTypeStr=boolean
  Bit3 : Inport  Port=4  OutDataTypeStr=boolean
  Bit4 : Inport  Port=5  OutDataTypeStr=boolean
  Bit5 : Inport  Port=6  OutDataTypeStr=boolean
  Bit6 : Inport  Port=7  OutDataTypeStr=boolean
  Bit7 : Inport  Port=8  OutDataTypeStr=boolean
  Bit Clear : simulink/Logic and Bit Operations/Bit Clear  iBit=0
      settings: SourceProductName=Simulink  SourceProductBaseCode=SL
  Bit Clear1 : simulink/Logic and Bit Operations/Bit Clear  iBit=1
      settings: SourceProductName=Simulink  SourceProductBaseCode=SL
  Bit Clear2 : simulink/Logic and Bit Operations/Bit Clear  iBit=2
      settings: SourceProductName=Simulink  SourceProductBaseCode=SL
  Bit Clear3 : simulink/Logic and Bit Operations/Bit Clear  iBit=3
      settings: SourceProductName=Simulink  SourceProductBaseCode=SL
  Bit Clear4 : simulink/Logic and Bit Operations/Bit Clear  iBit=5
      settings: SourceProductName=Simulink  SourceProductBaseCode=SL
  Bit Clear5 : simulink/Logic and Bit Operations/Bit Clear  iBit=4
      settings: SourceProductName=Simulink  SourceProductBaseCode=SL
  Bit Clear6 : simulink/Logic and Bit Operations/Bit Clear  iBit=6
      settings: SourceProductName=Simulink  SourceProductBaseCode=SL
  Bit Clear7 : simulink/Logic and Bit Operations/Bit Clear  iBit=7
      settings: SourceProductName=Simulink  SourceProductBaseCode=SL
  Bit Set : simulink/Logic and Bit Operations/Bit Set  iBit=0
      settings: SourceProductName=Simulink  SourceProductBaseCode=SL
  Bit Set1 : simulink/Logic and Bit Operations/Bit Set  iBit=1
      settings: SourceProductName=Simulink  SourceProductBaseCode=SL
  Bit Set2 : simulink/Logic and Bit Operations/Bit Set  iBit=2
      settings: SourceProductName=Simulink  SourceProductBaseCode=SL
  Bit Set3 : simulink/Logic and Bit Operations/Bit Set  iBit=3
      settings: SourceProductName=Simulink  SourceProductBaseCode=SL
  Bit Set4 : simulink/Logic and Bit Operations/Bit Set  iBit=4
      settings: SourceProductName=Simulink  SourceProductBaseCode=SL
  Bit Set5 : simulink/Logic and Bit Operations/Bit Set  iBit=5
      settings: SourceProductName=Simulink  SourceProductBaseCode=SL
  Bit Set6 : simulink/Logic and Bit Operations/Bit Set  iBit=6
      settings: SourceProductName=Simulink  SourceProductBaseCode=SL
  Bit Set7 : simulink/Logic and Bit Operations/Bit Set  iBit=7
      settings: SourceProductName=Simulink  SourceProductBaseCode=SL
  Delay : Delay  DelayLength=1  InitialCondition=0
  Switch{1..8} (8 alike) : Switch  Criteria=u2 > Threshold
  Index_8Bits : Outport  OutDataTypeStr=uint8
  wires:
  Bit Clear7/1 -> Switch8/3
  Bit Clear6/1 -> Switch7/3
  Bit Clear5/1 -> Switch5/3
  Bit Clear4/1 -> Switch6/3
  Bit Clear3/1 -> Switch4/3
  Bit Clear2/1 -> Switch3/3
  Bit Clear1/1 -> Switch2/3
  Bit Clear/1 -> Switch1/3
  Bit Set4/1 -> Switch5/1
  Bit Set2/1 -> Switch3/1
  Switch4/1 -> Bit Set4/1, Bit Clear5/1
  Switch6/1 -> Bit Set6/1, Bit Clear6/1
  Bit Set5/1 -> Switch6/1
  Switch7/1 -> Bit Set7/1, Bit Clear7/1
  Switch2/1 -> Bit Set2/1, Bit Clear2/1
  Bit Set3/1 -> Switch4/1
  Bit Set/1 -> Switch1/1
  Switch3/1 -> Bit Set3/1, Bit Clear3/1
  Bit6/1 -> Switch7/2
  Bit7/1 -> Switch8/2
  Bit Set6/1 -> Switch7/1
  Bit4/1 -> Switch5/2
  Bit5/1 -> Switch6/2
  Bit2/1 -> Switch3/2
  Bit Set1/1 -> Switch2/1
  Delay/1 -> Bit Set/1, Bit Clear/1
  Switch5/1 -> Bit Set5/1, Bit Clear4/1
  Bit1/1 -> Switch2/2
  Switch1/1 -> Bit Set1/1, Bit Clear1/1
  Switch8/1 -> Delay/1, Index_8Bits/1
  Bit3/1 -> Switch4/2
  Bit0/1 -> Switch1/2
  Bit Set7/1 -> Switch8/1

== system ADIA/ADAS_Diagnostics/Diagnostics_Processing/DTC_ACC_Accel_Decel_Safety_Violation/Latch  ==
  Input : Inport
  Latch Reset : Inport  Port=2
  Constant11 : Constant  Value=0  OutDataTypeStr=Inherit: Inherit via back propagation
  Constant12 : Constant  OutDataTypeStr=Inherit: Inherit via back propagation
  Switch : Switch  Threshold=1  OutDataTypeStr=Inherit: Inherit via back propagation  SaturateOnIntegerOverflow=on  InputSameDT=on
  Switch1 : Switch  Threshold=1  OutDataTypeStr=Inherit: Inherit via back propagation  SaturateOnIntegerOverflow=on  InputSameDT=on
  Unit Delay1 : UnitDelay  SampleTime=-1
  Output : Outport  InitialOutput=0
  wires:
  Switch1/1 -> Switch/3
  Latch Reset/1 -> Switch/2
  Switch/1 -> Output/1, Unit Delay1/1
  Unit Delay1/1 -> Switch1/3
  Input/1 -> Switch1/2
  Constant11/1 -> Switch/1
  Constant12/1 -> Switch1/1

== system ADIA/ADAS_Diagnostics/Diagnostics_Processing/DTC_ACC_Accel_Decel_Safety_Violation/Latch 1 ==
  Input : Inport
  Latch Reset : Inport  Port=2
  Constant11 : Constant  Value=0  OutDataTypeStr=Inherit: Inherit via back propagation
  Constant12 : Constant  OutDataTypeStr=Inherit: Inherit via back propagation
  Switch : Switch  Threshold=1  OutDataTypeStr=Inherit: Inherit via back propagation  SaturateOnIntegerOverflow=on  InputSameDT=on
  Switch1 : Switch  Threshold=1  OutDataTypeStr=Inherit: Inherit via back propagation  SaturateOnIntegerOverflow=on  InputSameDT=on
  Unit Delay1 : UnitDelay  SampleTime=-1
  Output : Outport  InitialOutput=0
  wires:
  Constant12/1 -> Switch1/1
  Constant11/1 -> Switch/1
  Input/1 -> Switch1/2
  Unit Delay1/1 -> Switch1/3
  Switch/1 -> Unit Delay1/1, Output/1
  Latch Reset/1 -> Switch/2
  Switch1/1 -> Switch/3

== system ADIA/ADAS_Diagnostics/Diagnostics_Processing/DTC_ACC_Accel_Decel_Safety_Violation/Timer1 ==
  incrcondition : Inport
  incrvalue : Inport  Port=2
  decr condition : Inport  Port=3
  decvalue : Inport  Port=4
  maxlimit : Inport  Port=5
  reset : Inport  Port=6
  Constant{,1..3} (4 alike) : Constant  Value=0  OutDataTypeStr=Inherit: Inherit via back propagation
  MinMax1 : MinMax  Inputs=2  OutDataTypeStr=Inherit: Inherit via back propagation  InputSameDT=on
  MinMax2 : MinMax  Function=max  Inputs=2  OutDataTypeStr=Inherit: Inherit via back propagation  InputSameDT=on
  Relational Operator : RelationalOperator  OutDataTypeStr=boolean  RndMeth=Nearest
  Sum : Sum  Inputs=++-  OutDataTypeStr=Inherit: Inherit via back propagation  InputSameDT=on
  Unit Delay : UnitDelay  SampleTime=-1
  dec switch : Switch  Criteria=u2 ~= 0  Threshold=1  OutDataTypeStr=Inherit: Inherit via back propagation  InputSameDT=on
  inc switch : Switch  Criteria=u2 ~= 0  Threshold=1  OutDataTypeStr=Inherit: Inherit via back propagation  InputSameDT=on
  reset switch : Switch  Criteria=u2 ~= 0  Threshold=1  OutDataTypeStr=Inherit: Inherit via back propagation  InputSameDT=on
  counter out : Outport
  counter_status : Outport  Port=2
  wires:
  incrcondition/1 -> inc switch/2
  decr condition/1 -> dec switch/2
  Constant1/1 -> dec switch/3
  dec switch/1 -> Sum/3
  MinMax1/1 -> reset switch/3
  incrvalue/1 -> inc switch/1
  MinMax2/1 -> MinMax1/1
  Constant/1 -> inc switch/3
  reset/1 -> reset switch/2
  Unit Delay/1 -> Sum/1
  reset switch/1 -> Unit Delay/1, Relational Operator/1, counter out/1
  Constant2/1 -> MinMax2/1
  maxlimit/1 -> Relational Operator/2, MinMax1/2
  Sum/1 -> MinMax2/2
  inc switch/1 -> Sum/2
  Constant3/1 -> reset switch/1
  Relational Operator/1 -> counter_status/1
  decvalue/1 -> dec switch/1

== system ADIA/ADAS_Diagnostics/Diagnostics_Processing/DTC_ACC_Accel_Decel_Safety_Violation/Timer2 ==
  incrcondition : Inport
  incrvalue : Inport  Port=2
  decr condition : Inport  Port=3
  decvalue : Inport  Port=4
  maxlimit : Inport  Port=5
  reset : Inport  Port=6
  Constant{,1..3} (4 alike) : Constant  Value=0  OutDataTypeStr=Inherit: Inherit via back propagation
  MinMax1 : MinMax  Inputs=2  OutDataTypeStr=Inherit: Inherit via back propagation  InputSameDT=on
  MinMax2 : MinMax  Function=max  Inputs=2  OutDataTypeStr=Inherit: Inherit via back propagation  InputSameDT=on
  Relational Operator : RelationalOperator  OutDataTypeStr=boolean  RndMeth=Nearest
  Sum : Sum  Inputs=++-  OutDataTypeStr=Inherit: Inherit via back propagation  InputSameDT=on
  Unit Delay : UnitDelay  SampleTime=-1
  dec switch : Switch  Criteria=u2 ~= 0  Threshold=1  OutDataTypeStr=Inherit: Inherit via back propagation  InputSameDT=on
  inc switch : Switch  Criteria=u2 ~= 0  Threshold=1  OutDataTypeStr=Inherit: Inherit via back propagation  InputSameDT=on
  reset switch : Switch  Criteria=u2 ~= 0  Threshold=1  OutDataTypeStr=Inherit: Inherit via back propagation  InputSameDT=on
  counter out : Outport
  counter_status : Outport  Port=2
  wires:
  decvalue/1 -> dec switch/1
  Relational Operator/1 -> counter_status/1
  Constant3/1 -> reset switch/1
  inc switch/1 -> Sum/2
  Sum/1 -> MinMax2/2
  maxlimit/1 -> MinMax1/2, Relational Operator/2
  Constant2/1 -> MinMax2/1
  reset switch/1 -> counter out/1, Relational Operator/1, Unit Delay/1
  Unit Delay/1 -> Sum/1
  reset/1 -> reset switch/2
  Constant/1 -> inc switch/3
  MinMax2/1 -> MinMax1/1
  incrvalue/1 -> inc switch/1
  MinMax1/1 -> reset switch/3
  dec switch/1 -> Sum/3
  Constant1/1 -> dec switch/3
  decr condition/1 -> dec switch/2
  incrcondition/1 -> inc switch/2

== system ADIA/ADAS_Diagnostics/Diagnostics_Processing/DTC_ACC_Displacement_Safety_Violation/Counter ==
  ADIAve_g_ESC_VeSpd : Inport  OutDataTypeStr=single  PortDimensions=1
  maxlimit : Inport  Port=2
  Enable : EnablePort  StatesWhenEnabling=reset
  Constant1 : Constant  Value=mps_to_kph
  Constant2 : Constant  Value=0  OutDataTypeStr=Inherit: Inherit via back propagation
  Constant4 : Constant  Value=SYS_dT20ms
  Divide : Product  Inputs=*/
  Divide1 : Product  Inputs=**
  MinMax1 : MinMax  Inputs=2  OutDataTypeStr=Inherit: Inherit via back propagation  InputSameDT=on
  MinMax2 : MinMax  Function=max  Inputs=2  OutDataTypeStr=Inherit: Inherit via back propagation  InputSameDT=on
  Relational Operator : RelationalOperator  OutDataTypeStr=boolean  RndMeth=Nearest
  Sum : Sum  OutDataTypeStr=Inherit: Inherit via back propagation  InputSameDT=on
  Unit Delay : UnitDelay  SampleTime=-1
  counter out : Outport
  counter_status : Outport  Port=2
  wires:
  MinMax2/1 -> MinMax1/1
  Unit Delay/1 -> Sum/1
  MinMax1/1 -> Relational Operator/1, Unit Delay/1, counter out/1
  Constant2/1 -> MinMax2/1
  maxlimit/1 -> Relational Operator/2, MinMax1/2
  Sum/1 -> MinMax2/2
  Divide1/1 -> Sum/2
  Relational Operator/1 -> counter_status/1
  Constant4/1 -> Divide1/2
  ADIAve_g_ESC_VeSpd/1 -> Divide/1
  Constant1/1 -> Divide/2
  Divide/1 -> Divide1/1

== system ADIA/ADAS_Diagnostics/Diagnostics_Processing/DTC_ACC_Displacement_Safety_Violation/Latch 2 ==
  Input : Inport
  Latch Reset : Inport  Port=2
  Constant11 : Constant  Value=0  OutDataTypeStr=Inherit: Inherit via back propagation
  Constant12 : Constant  OutDataTypeStr=Inherit: Inherit via back propagation
  Switch : Switch  Threshold=1  OutDataTypeStr=Inherit: Inherit via back propagation  SaturateOnIntegerOverflow=on  InputSameDT=on
  Switch1 : Switch  Threshold=1  OutDataTypeStr=Inherit: Inherit via back propagation  SaturateOnIntegerOverflow=on  InputSameDT=on
  Unit Delay1 : UnitDelay  SampleTime=-1
  Output : Outport  InitialOutput=0
  wires:
  Switch1/1 -> Switch/3
  Latch Reset/1 -> Switch/2
  Switch/1 -> Output/1, Unit Delay1/1
  Unit Delay1/1 -> Switch1/3
  Input/1 -> Switch1/2
  Constant11/1 -> Switch/1
  Constant12/1 -> Switch1/1

== system ADIA/ADAS_Diagnostics/Diagnostics_Processing/DTC_ACC_Displacement_Safety_Violation/Timer1 ==
  incrcondition : Inport
  incrvalue : Inport  Port=2
  decr condition : Inport  Port=3
  decvalue : Inport  Port=4
  maxlimit : Inport  Port=5
  reset : Inport  Port=6
  Constant{,1..3} (4 alike) : Constant  Value=0  OutDataTypeStr=Inherit: Inherit via back propagation
  MinMax1 : MinMax  Inputs=2  OutDataTypeStr=Inherit: Inherit via back propagation  InputSameDT=on
  MinMax2 : MinMax  Function=max  Inputs=2  OutDataTypeStr=Inherit: Inherit via back propagation  InputSameDT=on
  Relational Operator : RelationalOperator  OutDataTypeStr=boolean  RndMeth=Nearest
  Sum : Sum  Inputs=++-  OutDataTypeStr=Inherit: Inherit via back propagation  InputSameDT=on
  Unit Delay : UnitDelay  SampleTime=-1
  dec switch : Switch  Criteria=u2 ~= 0  Threshold=1  OutDataTypeStr=Inherit: Inherit via back propagation  InputSameDT=on
  inc switch : Switch  Criteria=u2 ~= 0  Threshold=1  OutDataTypeStr=Inherit: Inherit via back propagation  InputSameDT=on
  reset switch : Switch  Criteria=u2 ~= 0  Threshold=1  OutDataTypeStr=Inherit: Inherit via back propagation  InputSameDT=on
  counter out : Outport
  counter_status : Outport  Port=2
  wires:
  decvalue/1 -> dec switch/1
  Relational Operator/1 -> counter_status/1
  Constant3/1 -> reset switch/1
  inc switch/1 -> Sum/2
  Sum/1 -> MinMax2/2
  maxlimit/1 -> MinMax1/2, Relational Operator/2
  Constant2/1 -> MinMax2/1
  reset switch/1 -> counter out/1, Relational Operator/1, Unit Delay/1
  Unit Delay/1 -> Sum/1
  reset/1 -> reset switch/2
  Constant/1 -> inc switch/3
  MinMax2/1 -> MinMax1/1
  incrvalue/1 -> inc switch/1
  MinMax1/1 -> reset switch/3
  dec switch/1 -> Sum/3
  Constant1/1 -> dec switch/3
  decr condition/1 -> dec switch/2
  incrcondition/1 -> inc switch/2

== system ADIA/ADAS_Diagnostics/Diagnostics_Processing/DTC_ACC_HoldConfirm_Safety_Violation/Latch 2 ==
  Input : Inport
  Latch Reset : Inport  Port=2
  Constant11 : Constant  Value=0  OutDataTypeStr=Inherit: Inherit via back propagation
  Constant12 : Constant  OutDataTypeStr=Inherit: Inherit via back propagation
  Switch : Switch  Threshold=1  OutDataTypeStr=Inherit: Inherit via back propagation  SaturateOnIntegerOverflow=on  InputSameDT=on
  Switch1 : Switch  Threshold=1  OutDataTypeStr=Inherit: Inherit via back propagation  SaturateOnIntegerOverflow=on  InputSameDT=on
  Unit Delay1 : UnitDelay  SampleTime=-1
  Output : Outport  InitialOutput=0
  wires:
  Constant12/1 -> Switch1/1
  Constant11/1 -> Switch/1
  Input/1 -> Switch1/2
  Unit Delay1/1 -> Switch1/3
  Switch/1 -> Unit Delay1/1, Output/1
  Latch Reset/1 -> Switch/2
  Switch1/1 -> Switch/3
